simulink model "airspeed_from_throttle_loop"  (Simulink 7.4)
settings: Solver=ode45  StartTime=0.0  StopTime=100  RelTol=1e-3
values from neighbouring files (symbols this model uses):
  a_Vt1 = den(2)    [computeGains.m]
  a_Vt2 = num(2)    [computeGains.m]
  P = varargin{5}    [my_mav_dynamics.m]
settings Model: Creator=beard  LastModifiedBy=beard

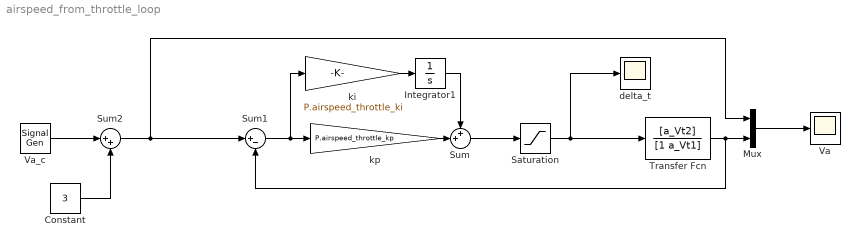
== system airspeed_from_throttle_loop ==
  Constant : Constant  Value=3  OutDataType=fixdt(1, 16)  OutScaling=2^0
  Integrator1 : Integrator
  Mux : Mux  Inputs=2
  Saturation : Saturate  UpperLimit=1  LowerLimit=0  OutDataType=fixdt(1, 16)  OutScaling=2^0
  Sum : Sum  Inputs=++|  OutDataType=fixdt(1, 16)  OutScaling=2^0
  Sum1 : Sum  Inputs=|+-  OutDataType=fixdt(1, 16)  OutScaling=2^0
  Sum2 : Sum  Inputs=|++  OutDataType=fixdt(1, 16)  OutScaling=2^0
  Transfer Fcn : TransferFcn  Numerator=[a_Vt2]  Denominator=[1 a_Vt1]
  Va : Scope
      settings: TimeRange=100  YMin=-3  YMax=3
  Va_c : SignalGenerator  WaveForm=square  Amplitude=2  Frequency=.02
  delta_t : Scope
      settings: TimeRange=100  YMin=-3  YMax=3
  ki : Gain  Gain=P.airspeed_throttle_ki  ParameterDataType=fixdt(1, 16)  ParameterScaling=2^0  OutDataType=fixdt(1, 16)  OutScaling=2^0
  kp : Gain  Gain=P.airspeed_throttle_kp  ParameterDataType=fixdt(1, 16)  ParameterScaling=2^0  OutDataType=fixdt(1, 16)  OutScaling=2^0
  wires:
  Sum/1 -> Saturation/1
  kp/1 -> Sum/2
  Sum1/1 -> kp/1, ki/1
  ki/1 -> Integrator1/1
  Integrator1/1 -> Sum/1
  Mux/1 -> Va/1
  Transfer Fcn/1 -> Mux/2, Sum1/2
  Saturation/1 -> Transfer Fcn/1, delta_t/1
  Va_c/1 -> Sum2/1
  Constant/1 -> Sum2/2
  Sum2/1 -> Sum1/1, Mux/1
